simulink model "test"  (R2017a)
settings: Solver=VariableStepAuto  StartTime=0.0  StopTime=20.0  MaxStep=0.01  RelTol=1e-3
settings Model: Creator=HP  LastModifiedBy=HP

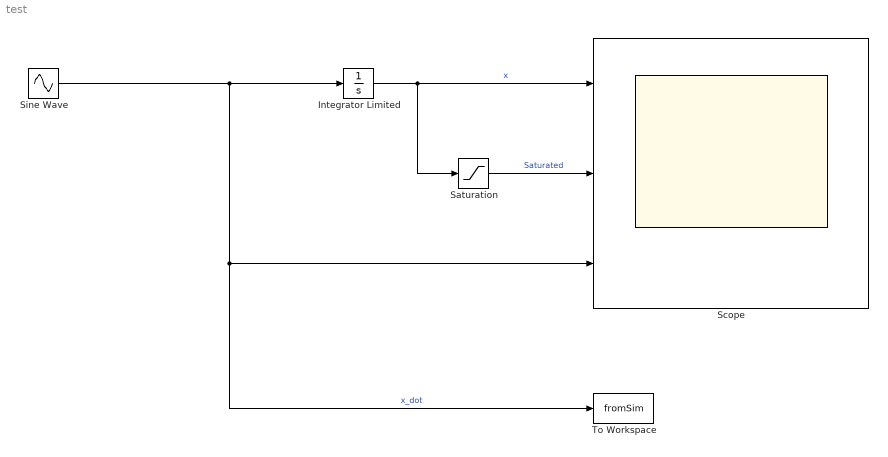
== system test ==
  Integrator Limited : Integrator  LimitOutput=on  UpperSaturationLimit=0.5  LowerSaturationLimit=-0.5
      settings: AttributesFormatString=|
      | %<BlockType>
      | %<InitialCondition>
  Saturation : Saturate  UpperLimit=0.25  LowerLimit=-0.25
  Scope : Scope  NumInputPorts=3
  Sine Wave : Sin  SampleTime=0
  To Workspace : ToWorkspace  VariableName=fromSim  SampleTime=-1
  wires:
  Sine Wave/1 -> To Workspace/1, Scope/3, Integrator Limited/1  "x_dot"
  Integrator Limited/1 -> Saturation/1, Scope/1  "x"
  Saturation/1 -> Scope/2  "Saturated"
